simulink model "Linear_Moving_Setpoint_FF"  (R2020b)
settings: Solver=VariableStepAuto  StartTime=0.0  StopTime=t_sim  RelTol=1e-3
undefined symbols (not defined in the file): A1_sim, B1_sim, C1_setp_ctrl, des_traj_handle, FF_act_handle, K1, KI, KP, r_sim, SP_sel, x1_0
libraries: simulink x1
settings Model: Creator=domin  LastModifiedBy=domin

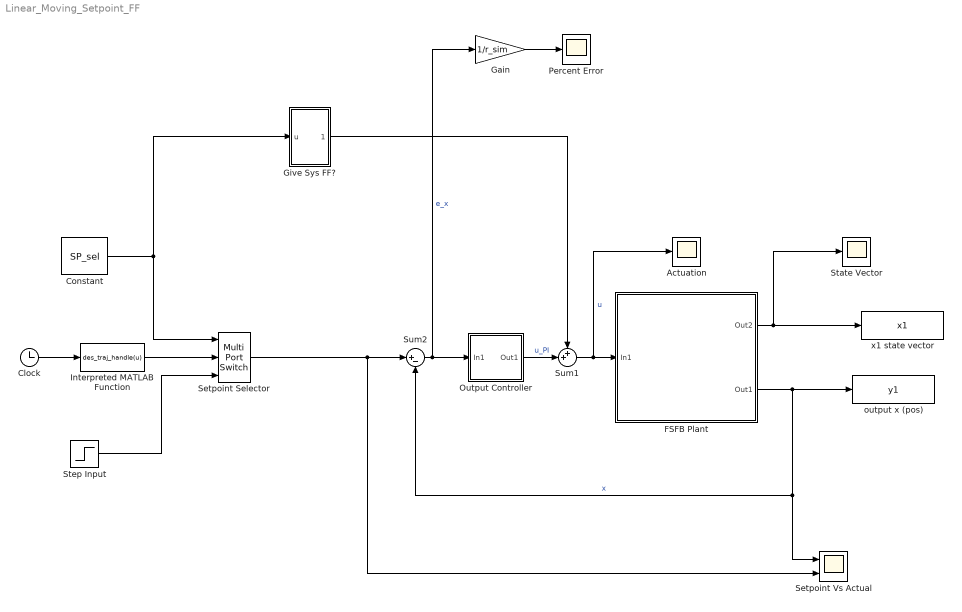
== system Linear_Moving_Setpoint_FF ==
  Actuation : Scope
  Clock : Clock
  Constant : Constant  Value=SP_sel
  FSFB Plant : Subsystem
  Gain : Gain  Gain=1/r_sim
  Give Sys FF? : Subsystem
  Interpreted MATLAB Function : MATLABFcn  MATLABFcn=des_traj_handle(u)
  Output Controller : Subsystem
  Percent Error : Scope
  Setpoint Selector : MultiPortSwitch  Inputs=2
  Setpoint Vs Actual : Scope  NumInputPorts=2
  State Vector : Scope
  Step Input : Step  After=r_sim  SampleTime=0
  Sum1 : Sum  Inputs=++|
  Sum2 : Sum  Inputs=|+-
  output x (pos) : ToWorkspace  VariableName=y1  SampleTime=-1
  x1 state vector : ToWorkspace  VariableName=x1  SampleTime=-1
  wires:
  Sum2/1 -> Output Controller/1(In1), Gain/1  "e_x"
  FSFB Plant/2(Out1) -> Sum2/2, Setpoint Vs Actual/1, output x (pos)/1  "x"
  Output Controller/1(Out1) -> Sum1/2  "u_PI"
  FSFB Plant/1(Out2) -> x1 state vector/1, State Vector/1
  Gain/1 -> Percent Error/1
  Setpoint Selector/1 -> Setpoint Vs Actual/2, Sum2/1
  Interpreted MATLAB Function/1 -> Setpoint Selector/2
  Step Input/1 -> Setpoint Selector/3
  Constant/1 -> Setpoint Selector/1, Give Sys FF?/1(u)
  Sum1/1 -> Actuation/1, FSFB Plant/1(In1)  "u"
  Give Sys FF?/1(Out1) -> Sum1/1
  Clock/1 -> Interpreted MATLAB Function/1

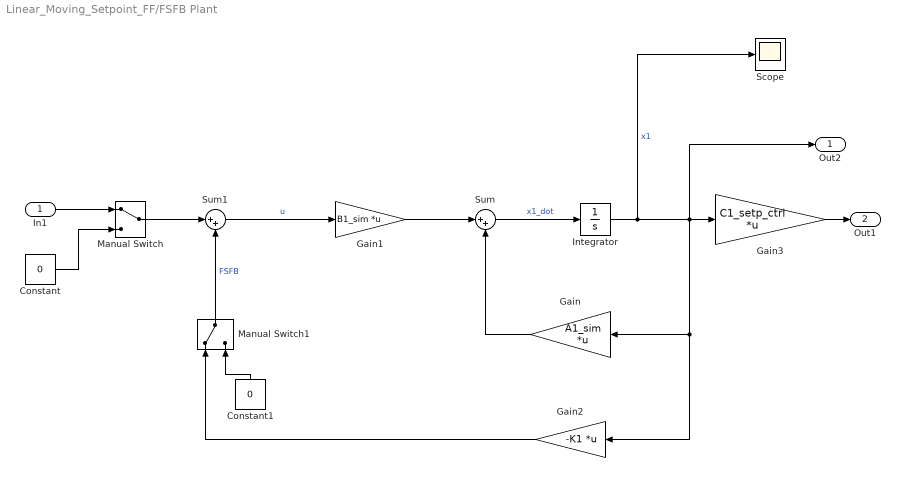
== system Linear_Moving_Setpoint_FF/FSFB Plant ==
  In1 : Inport
  Constant : Constant  Value=0
  Constant1 : Constant  Value=0
  Gain : Gain  Gain=A1_sim  Multiplication=Matrix(K*u)
  Gain1 : Gain  Gain=B1_sim  Multiplication=Matrix(K*u)
  Gain2 : Gain  Gain=-K1  Multiplication=Matrix(K*u)
  Gain3 : Gain  Gain=C1_setp_ctrl  Multiplication=Matrix(K*u)
  Integrator : Integrator  InitialCondition=x1_0
  Manual Switch : ManualSwitch
  Manual Switch1 : ManualSwitch
  Scope : Scope
  Sum : Sum  Inputs=|++
  Sum1 : Sum  Inputs=|++
  Out2 : Outport
  Out1 : Outport  Port=2
  wires:
  Gain1/1 -> Sum/1
  Sum/1 -> Integrator/1  "x1_dot"
  Integrator/1 -> Scope/1, Out2/1, Gain2/1, Gain/1, Gain3/1  "x1"
  Gain3/1 -> Out1/1
  Gain/1 -> Sum/2
  In1/1 -> Manual Switch/1
  Constant/1 -> Manual Switch/2
  Sum1/1 -> Gain1/1  "u"
  Gain2/1 -> Manual Switch1/1
  Manual Switch/1 -> Sum1/1
  Manual Switch1/1 -> Sum1/2  "FSFB"
  Constant1/1 -> Manual Switch1/2

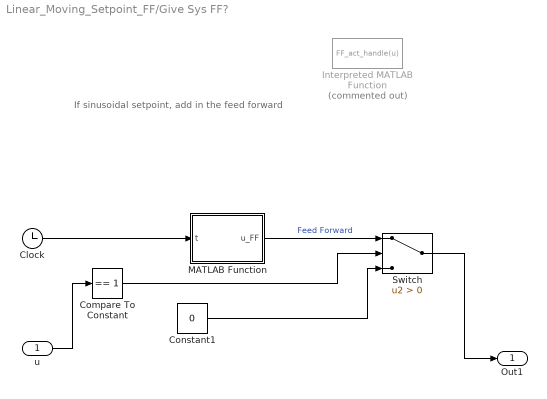
== system Linear_Moving_Setpoint_FF/Give Sys FF? ==
  note: If sinusoidal setpoint, add in the feed forward
  u : Inport
  Clock : Clock
  Compare To Constant : simulink/Logic and Bit Operations/Compare To Constant  relop===  const=1  OutDataTypeStr=boolean
  Constant1 : Constant  Value=0
  Interpreted MATLAB Function : MATLABFcn  Commented=on  MATLABFcn=FF_act_handle(u)
  MATLAB Function : MATLAB Function  TreatAsAtomicUnit=on
  Switch : Switch  Criteria=u2 > Threshold
  Out1 : Outport
  wires:
  Switch/1 -> Out1/1
  u/1 -> Compare To Constant/1
  MATLAB Function/1(u_FF) -> Switch/1  "Feed Forward"
  Compare To Constant/1 -> Switch/2
  Constant1/1 -> Switch/3
  Clock/1 -> MATLAB Function/1(t)

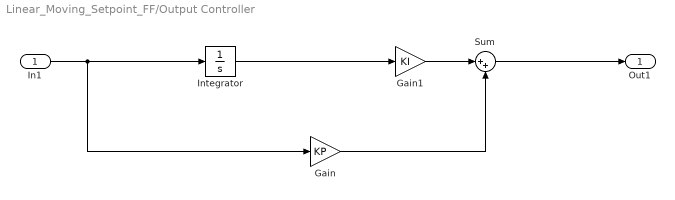
== system Linear_Moving_Setpoint_FF/Output Controller ==
  In1 : Inport
  Gain : Gain  Gain=KP
  Gain1 : Gain  Gain=KI
  Integrator : Integrator
  Sum : Sum  Inputs=|++
  Out1 : Outport
  wires:
  In1/1 -> Integrator/1, Gain/1
  Gain/1 -> Sum/2
  Gain1/1 -> Sum/1
  Sum/1 -> Out1/1
  Integrator/1 -> Gain1/1

== matlab function Linear_Moving_Setpoint_FF/Give Sys FF?/MATLAB Function ==
  data: t input; u_FF output
function u_FF = fcn(t)

u_FF = cos(t./4.0).*9.787113714149716e-1+sin(t./4.0).*3.700539911107918-...
    cosh(2.977146284615521e+2.*7.687987759523578e+7.*t.*5.379844734561511e-10).*...
    3.407512593157144-exp(t.*-2.0).*(cos(t./4.0)+sin(t./4.0).*1.678138930946272)....
    *1.097280108322348e-1-2.977146284615521e+2.*7.687987759523578e+7.*...
    sinh(2.977146284615521e+2.*7.687987759523578e+7.*t.*5.379844734561511e-10)....
    *1.173877768666137e-10;
